simulink model "benchmarkss"  (Simulink 7.9)
settings: Solver=ode15s  SolverMode=SingleTasking  StartTime=0.0  StopTime=150  FixedStep=0.01  RelTol=1e-5  AbsTol=1e-8
values from neighbouring files (symbols this model uses):
  Qin0 = 18446    [states.mat]
  Qintr = 16485.6074222    [states.mat]
  Qintrawstate = 0    [states.mat]
  Qintrintstate = -2014.39257785    [states.mat]
  SETTLERINIT = [12.501625291 18.1183173569 29.5480012161 69.0014901899 356.282470924 356.282470935 356.282470923 356.282470934 356.282470923 6399.29814462 30 30 ... (80 elements, 1x80)]    [states.mat]
  SO5awstate = 1160.56564631    [states.mat]
  SO5intstate = -1172.91424974    [states.mat]
  XINIT1 = [30 3.24393684526 1149.16825994 98.6028769556 2552.10953282 151.672059002 446.924884063 0.00769641505704 3.51326345277 11.8311788245 1.36208895519 6.17753127623 ... (15 elements, 1x15)]    [states.mat]
  XINIT2 = [30 1.67067015162 1149.16825989 91.7032143318 2552.3710778 151.530315219 448.083853672 6.02712619456e-05 0.999999999994 12.5481626127 0.788988192675 5.95370072728 ... (15 elements, 1x15)]    [states.mat]
  XINIT3 = [30 1.21951265626 1149.16825982 69.6593696369 2560.20249467 152.687333601 449.633569515 1.63502587307 6.22889933341 7.31965726619 0.830700760805 4.71313752465 ... (15 elements, 1x15)]    [states.mat]
  XINIT4 = [30 0.973258200881 1149.16825975 54.4484250888 2563.31043926 153.710829707 451.185250351 2.47452269527 11.0693154946 2.7825370247 0.752763867168 3.84029820267 ... (15 elements, 1x15)]    [states.mat]
  XINIT5 = [30 0.808007806448 1149.16825967 44.4828030813 2562.85141224 154.163014752 452.736701239 2.00000000001 13.5243173117 0.671926961295 0.66449772338 3.26046452657 ... (15 elements, 1x15)]    [states.mat]
  XINITDELAY = [1601328.22267 1310222.01149 61339852.2439 6069822.46695 135212240.468 8102155.18077 23793923.6941 69863.2148447 472426.142984 605627.248842 151411.673606 366699.347571 ... (15 elements, 1x15)]    [states.mat]
undefined symbols (not defined in the file or in its folder): carb1, carb2, carb3, carb4, carb5, DIM, Kfeedforward, KLa1, KLa2, KLa3, KLa4, KLa5_max, KLa5offset, KQintr, KSO5, LAYER, MODELTYPE, PAR1, PAR2, PAR3, PAR4, PAR5, Qffref, Qintr_max, Qintroffset, QintrT, SETTLERPAR, SNO2ref, SO5ref, SOSAT1, SOSAT2, SOSAT3, SOSAT4, SOSAT5, T, TiQintr, TiSO5, TtQintr, TtSO5, useantiwindupQintr, useantiwindupSO5, VOL1, VOL2, VOL3, VOL4, VOL5
libraries: simulink x3
settings Model: Creator=ielulf  LastModifiedBy=SCUT2  ExtModeTrigMode=oneshot  ExtModeArmWhenConnect=off  ExtModeAutoUpdateStatusClock=off
settings DataIOCC: LimitDataPoints=off  SaveOutput=off  TimeSaveName=t  SignalLoggingName=sigsOut  OutputTimes=[143:(1/96):150]
settings OptimizationCC: BlockReduction=off  BooleanDataType=off  InitFltsAndDblsToZero=on
settings DebuggingCC: AlgebraicLoopMsg=none  SaveWithParameterizedLinksMsg=none  SignalResolutionControl=TryResolveAllWithWarning  SolverPrmCheckMsg=none  InheritedTsInSrcMsg=none  MultiTaskDSMMsg=warning  MultiTaskCondExecSysMsg=none  FcnCallInpInsideContextMsg=Use local settings  UnconnectedOutputMsg=none  StrictBusMsg=None
settings HardwareCC: TargetUnknown=on
settings RTWCC: TemplateMakefile=grt_unix.tmf  IncludeERTFirstTime=on
settings GRTTargetCC: TargetFcnLib=ansi_tfl_tmw.mat  CombineOutputUpdateFcns=off  GRTInterface=on

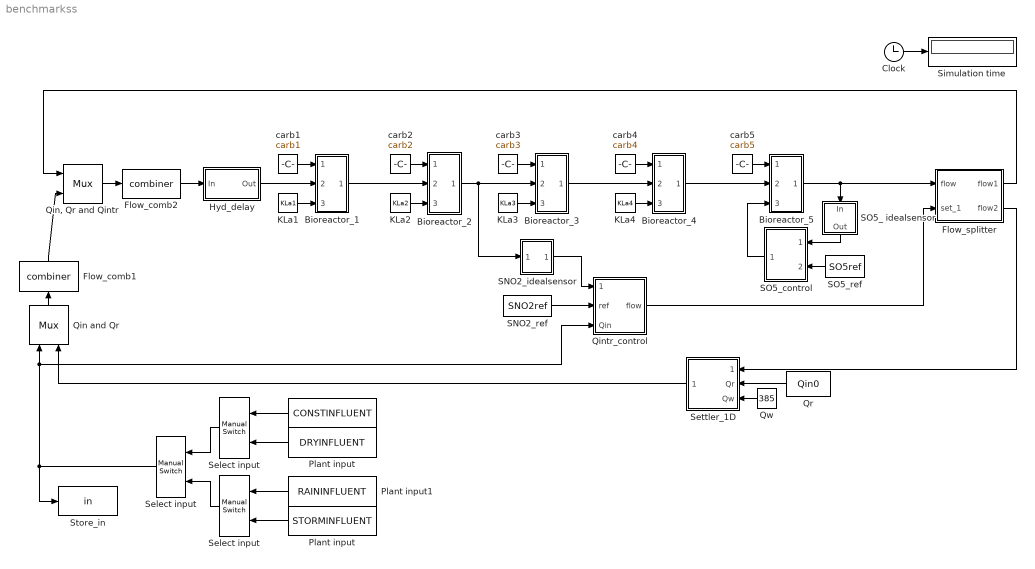
== system benchmarkss ==
  " " : FromWorkspace  VariableName=CONSTINFLUENT  OutputAfterFinalValue=Holding final value
  " Select input" : simulink/Signal Routing/Manual Switch  sw=1  action=0  varsize=off
  Bioreactor_1 : Subsystem
  Bioreactor_2 : Subsystem
  Bioreactor_3 : Subsystem
  Bioreactor_4 : Subsystem
  Bioreactor_5 : Subsystem
  Clock : Clock
  Flow_comb1 : S-Function  FunctionName=combiner  EnableBusSupport=off
  Flow_comb2 : S-Function  FunctionName=combiner  EnableBusSupport=off
  Flow_splitter : Subsystem
  Hyd_delay : Subsystem
  KLa1 : Constant  Value=KLa1
  KLa2 : Constant  Value=KLa2
  KLa3 : Constant  Value=KLa3
  KLa4 : Constant  Value=KLa4
  Plant input : FromWorkspace  VariableName=DRYINFLUENT  OutputAfterFinalValue=Holding final value
  "Plant input " : FromWorkspace  VariableName=STORMINFLUENT  OutputAfterFinalValue=Holding final value
  Plant input1 : FromWorkspace  VariableName=RAININFLUENT  OutputAfterFinalValue=Holding final value
  Qin and Qr : Mux  Inputs=2
  "Qin, Qr and Qintr" : Mux  Inputs=2
  Qintr_control : Subsystem
  Qr : Constant  Value=Qin0
  Qw : Constant  Value=385
  SNO2_idealsensor : Subsystem
  SNO2_ref : Constant  Value=SNO2ref
  SO5_ idealsensor : Subsystem
  SO5_control : Subsystem
  SO5_ref : Constant  Value=SO5ref
  Select input : simulink/Signal Routing/Manual Switch  sw=1  action=0  varsize=off
  "Select input " : simulink/Signal Routing/Manual Switch  sw=0  action=0  varsize=off
  Settler_1D : Subsystem
  Simulation time : Display
  Store_in : ToWorkspace  VariableName=in  SampleTime=-1
  carb1 : Constant  Value=carb1
  carb2 : Constant  Value=carb2
  carb3 : Constant  Value=carb3
  carb4 : Constant  Value=carb4
  carb5 : Constant  Value=carb5
  wires:
  Qin and Qr/1 -> Flow_comb1/1
  Flow_comb1/1 -> "Qin, Qr and Qintr"/2
  "Qin, Qr and Qintr"/1 -> Flow_comb2/1
  Flow_splitter/1(flow1) -> "Qin, Qr and Qintr"/1
  Settler_1D/1(output) -> Qin and Qr/2
  Qw/1 -> Settler_1D/3(Qw)
  Flow_splitter/2(flow2) -> Settler_1D/1(feed)
  Qr/1 -> Settler_1D/2(Qr)
  Bioreactor_5/1(out) -> Flow_splitter/1(flow), SO5_ idealsensor/1(In)
  Flow_comb2/1 -> Hyd_delay/1(In)
  Clock/1 -> Simulation time/1
  Plant input/1 -> Select input/2
  " "/1 -> Select input/1
  Hyd_delay/1(Out) -> Bioreactor_1/2(in)
  carb1/1 -> Bioreactor_1/1(carb)
  KLa1/1 -> Bioreactor_1/3(KLa)
  Bioreactor_1/1(out) -> Bioreactor_2/2(in)
  KLa2/1 -> Bioreactor_2/3(KLa)
  carb2/1 -> Bioreactor_2/1(carb)
  Bioreactor_2/1(out) -> Bioreactor_3/2(in), SNO2_idealsensor/1(In)
  KLa3/1 -> Bioreactor_3/3(KLa)
  carb3/1 -> Bioreactor_3/1(carb)
  Bioreactor_3/1(out) -> Bioreactor_4/2(in)
  KLa4/1 -> Bioreactor_4/3(KLa)
  carb4/1 -> Bioreactor_4/1(carb)
  Bioreactor_4/1(out) -> Bioreactor_5/2(in)
  carb5/1 -> Bioreactor_5/1(carb)
  Plant input1/1 -> "Select input "/1
  "Plant input "/1 -> "Select input "/2
  Select input/1 -> " Select input"/1
  "Select input "/1 -> " Select input"/2
  " Select input"/1 -> Store_in/1, Qin and Qr/1, Qintr_control/3(Qin)
  SNO2_ref/1 -> Qintr_control/2(ref)
  SNO2_idealsensor/1(Out) -> Qintr_control/1(meas)
  Qintr_control/1(flow) -> Flow_splitter/2(set_1)
  SO5_ref/1 -> SO5_control/2(O2_ref)
  SO5_control/1(KLa) -> Bioreactor_5/3(KLa)
  SO5_ idealsensor/1(Out) -> SO5_control/1(O2_meas)

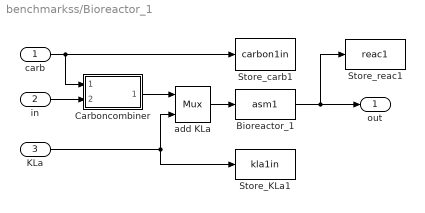
== system benchmarkss/Bioreactor_1 ==
  carb : Inport
  in : Inport  Port=2
  KLa : Inport  Port=3
  Bioreactor_1 : S-Function  FunctionName=asm1  Parameters=XINIT1,PAR1,VOL1,SOSAT1  EnableBusSupport=off
  Carboncombiner : Subsystem
  Store_KLa1 : ToWorkspace  VariableName=kla1in  SampleTime=-1
  Store_carb1 : ToWorkspace  VariableName=carbon1in  SampleTime=-1
  Store_reac1 : ToWorkspace  VariableName=reac1  SampleTime=-1
  add KLa : Mux  Inputs=2
  out : Outport
  wires:
  add KLa/1 -> Bioreactor_1/1
  Bioreactor_1/1 -> out/1, Store_reac1/1
  Carboncombiner/1(Output) -> add KLa/1
  carb/1 -> Store_carb1/1, Carboncombiner/1(C_flow)
  in/1 -> Carboncombiner/2(Input)
  KLa/1 -> add KLa/2, Store_KLa1/1

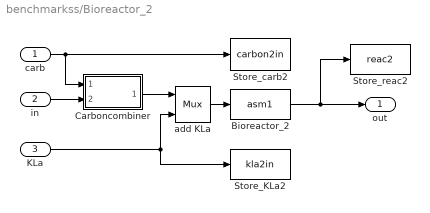
== system benchmarkss/Bioreactor_2 ==
  carb : Inport
  in : Inport  Port=2
  KLa : Inport  Port=3
  Bioreactor_2 : S-Function  FunctionName=asm1  Parameters=XINIT2,PAR2,VOL2,SOSAT2  EnableBusSupport=off
  Carboncombiner : Subsystem
  Store_KLa2 : ToWorkspace  VariableName=kla2in  SampleTime=-1
  Store_carb2 : ToWorkspace  VariableName=carbon2in  SampleTime=-1
  Store_reac2 : ToWorkspace  VariableName=reac2  SampleTime=-1
  add KLa : Mux  Inputs=2
  out : Outport
  wires:
  Bioreactor_2/1 -> out/1, Store_reac2/1
  add KLa/1 -> Bioreactor_2/1
  Carboncombiner/1(Output) -> add KLa/1
  carb/1 -> Carboncombiner/1(C_flow), Store_carb2/1
  in/1 -> Carboncombiner/2(Input)
  KLa/1 -> add KLa/2, Store_KLa2/1

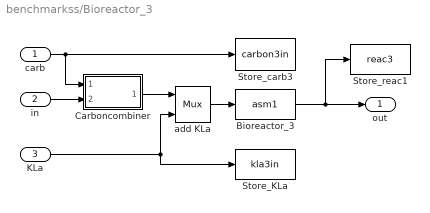
== system benchmarkss/Bioreactor_3 ==
  carb : Inport
  in : Inport  Port=2
  KLa : Inport  Port=3
  Bioreactor_3 : S-Function  FunctionName=asm1  Parameters=XINIT3,PAR3,VOL3,SOSAT3  EnableBusSupport=off
  Carboncombiner : Subsystem
  Store_KLa : ToWorkspace  VariableName=kla3in  SampleTime=-1
  Store_carb3 : ToWorkspace  VariableName=carbon3in  SampleTime=-1
  Store_reac1 : ToWorkspace  VariableName=reac3  SampleTime=-1
  add KLa : Mux  Inputs=2
  out : Outport
  wires:
  Bioreactor_3/1 -> out/1, Store_reac1/1
  add KLa/1 -> Bioreactor_3/1
  Carboncombiner/1(Output) -> add KLa/1
  carb/1 -> Carboncombiner/1(C_flow), Store_carb3/1
  in/1 -> Carboncombiner/2(Input)
  KLa/1 -> add KLa/2, Store_KLa/1

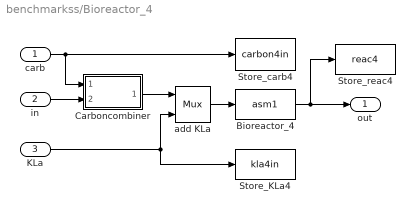
== system benchmarkss/Bioreactor_4 ==
  carb : Inport
  in : Inport  Port=2
  KLa : Inport  Port=3
  Bioreactor_4 : S-Function  FunctionName=asm1  Parameters=XINIT4,PAR4,VOL4,SOSAT4  EnableBusSupport=off
  Carboncombiner : Subsystem
  Store_KLa4 : ToWorkspace  VariableName=kla4in  SampleTime=-1
  Store_carb4 : ToWorkspace  VariableName=carbon4in  SampleTime=-1
  Store_reac4 : ToWorkspace  VariableName=reac4  SampleTime=-1
  add KLa : Mux  Inputs=2
  out : Outport
  wires:
  Bioreactor_4/1 -> out/1, Store_reac4/1
  add KLa/1 -> Bioreactor_4/1
  Carboncombiner/1(Output) -> add KLa/1
  carb/1 -> Carboncombiner/1(C_flow), Store_carb4/1
  in/1 -> Carboncombiner/2(Input)
  KLa/1 -> add KLa/2, Store_KLa4/1

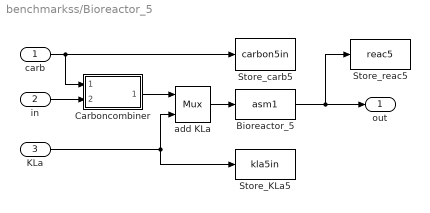
== system benchmarkss/Bioreactor_5 ==
  carb : Inport
  in : Inport  Port=2
  KLa : Inport  Port=3
  Bioreactor_5 : S-Function  FunctionName=asm1  Parameters=XINIT5,PAR5,VOL5,SOSAT5  EnableBusSupport=off
  Carboncombiner : Subsystem
  Store_KLa5 : ToWorkspace  VariableName=kla5in  SampleTime=-1
  Store_carb5 : ToWorkspace  VariableName=carbon5in  SampleTime=-1
  Store_reac5 : ToWorkspace  VariableName=reac5  SampleTime=-1
  add KLa : Mux  Inputs=2
  out : Outport
  wires:
  Bioreactor_5/1 -> out/1, Store_reac5/1
  add KLa/1 -> Bioreactor_5/1
  Carboncombiner/1(Output) -> add KLa/1
  carb/1 -> Carboncombiner/1(C_flow), Store_carb5/1
  in/1 -> Carboncombiner/2(Input)
  KLa/1 -> add KLa/2, Store_KLa5/1

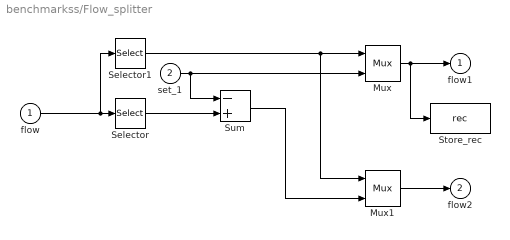
== system benchmarkss/Flow_splitter ==
  flow : Inport
  set_1 : Inport  Port=2
  Mux : Mux  Inputs=2
  Mux1 : Mux  Inputs=2
  Selector : Selector  InputPortWidth=15  IndexOptions=Index vector (dialog)  Indices=[15]  OutputSizes=1
  Selector1 : Selector  InputPortWidth=15  IndexOptions=Index vector (dialog)  Indices=[1 2 3 4 5 6 7 8 9 10 11 12 13 14]  OutputSizes=1
  Store_rec : ToWorkspace  VariableName=rec  SampleTime=-1
  Sum : Sum  Inputs=-+  SaturateOnIntegerOverflow=on  InputSameDT=on  OutDataTypeStr=Inherit: Same as first input
  flow1 : Outport
  flow2 : Outport  Port=2
  wires:
  flow/1 -> Selector1/1, Selector/1
  Mux/1 -> flow1/1, Store_rec/1
  Mux1/1 -> flow2/1
  set_1/1 -> Mux/2, Sum/1
  Selector/1 -> Sum/2
  Sum/1 -> Mux1/2
  Selector1/1 -> Mux/1, Mux1/1

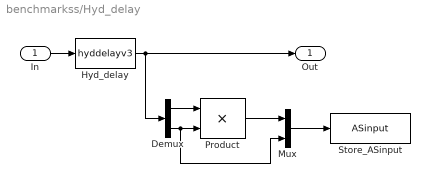
== system benchmarkss/Hyd_delay ==
  In : Inport
  Demux : Demux  Outputs=[14,1]
  Hyd_delay : S-Function  FunctionName=hyddelayv3  Parameters=XINITDELAY,PAR1,T  EnableBusSupport=off
  Mux : Mux  Inputs=2
  Product : Product  SaturateOnIntegerOverflow=on  OutDataTypeStr=Inherit: Same as first input
  Store_ASinput : ToWorkspace  VariableName=ASinput  SampleTime=-1
  Out : Outport
  wires:
  In/1 -> Hyd_delay/1
  Hyd_delay/1 -> Out/1, Demux/1
  Demux/1 -> Product/1
  Demux/2 -> Product/2, Mux/2
  Product/1 -> Mux/1
  Mux/1 -> Store_ASinput/1

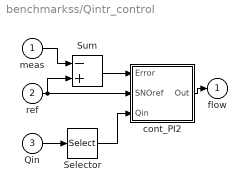
== system benchmarkss/Qintr_control ==
  meas : Inport
  ref : Inport  Port=2
  Qin : Inport  Port=3
  Selector : Selector  InputPortWidth=15  IndexOptions=Index vector (dialog)  Indices=[15]  OutputSizes=1
  Sum : Sum  Inputs=-+  SaturateOnIntegerOverflow=on  InputSameDT=on  OutDataTypeStr=Inherit: Same as first input
  cont_PI2 : Subsystem
  flow : Outport
  wires:
  Selector/1 -> cont_PI2/3(Qin)
  ref/1 -> cont_PI2/2(SNOref), Sum/2
  Qin/1 -> Selector/1
  cont_PI2/1(Out) -> flow/1
  Sum/1 -> cont_PI2/1(Error)
  meas/1 -> Sum/1

== system benchmarkss/SNO2_idealsensor ==
  In : Inport
  Mux : Mux  Inputs=6
  Selector : Selector  InputPortWidth=15  IndexOptions=Index vector (dialog)  Indices=[9]  OutputSizes=1
  To Workspace : ToWorkspace  VariableName=SNO2sensor  SampleTime=-1
  Out : Outport
  wires:
  Selector/1 -> Mux/3, Mux/4, Out/1, Mux/5, Mux/6, Mux/2, Mux/1
  In/1 -> Selector/1
  Mux/1 -> To Workspace/1

== system benchmarkss/SO5_ idealsensor ==
  In : Inport
  Mux : Mux  Inputs=6
  Selector : Selector  InputPortWidth=15  IndexOptions=Index vector (dialog)  Indices=[8]  OutputSizes=1
  To Workspace : ToWorkspace  VariableName=SO5sensor  SampleTime=-1
  Out : Outport
  wires:
  Selector/1 -> Mux/3, Mux/4, Out/1, Mux/5, Mux/6, Mux/2, Mux/1
  In/1 -> Selector/1
  Mux/1 -> To Workspace/1

== system benchmarkss/SO5_control ==
  O2_meas : Inport
  O2_ref : Inport  Port=2
  Sum : Sum  Inputs=-+  SaturateOnIntegerOverflow=on  InputSameDT=on  OutDataTypeStr=Inherit: Same as first input
  cont_PI : Subsystem
  KLa : Outport
  wires:
  O2_meas/1 -> Sum/1
  cont_PI/1(Out) -> KLa/1
  O2_ref/1 -> Sum/2
  Sum/1 -> cont_PI/1(In)

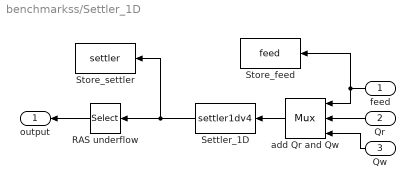
== system benchmarkss/Settler_1D ==
  feed : Inport
  Qr : Inport  Port=2
  Qw : Inport  Port=3
  RAS underflow : Selector  InputPortWidth=113  IndexOptions=Index vector (dialog)  Indices=[1 2 3 4 5 6 7 8 9 10 11 12 13 14 15]  OutputSizes=1
  Settler_1D : S-Function  FunctionName=settler1dv4  Parameters=SETTLERINIT,SETTLERPAR,DIM,LAYER,MODELTYPE  EnableBusSupport=off
  Store_feed : ToWorkspace  VariableName=feed  SampleTime=-1
  Store_settler : ToWorkspace  VariableName=settler  SampleTime=-1
  add Qr and Qw : Mux  Inputs=3
  output : Outport
  wires:
  add Qr and Qw/1 -> Settler_1D/1
  Qr/1 -> add Qr and Qw/2
  Qw/1 -> add Qr and Qw/3
  feed/1 -> add Qr and Qw/1, Store_feed/1
  RAS underflow/1 -> output/1
  Settler_1D/1 -> RAS underflow/1, Store_settler/1

== system benchmarkss/Bioreactor_1/Carboncombiner ==
  C_flow : Inport
  Input : Inport  Port=2
  Carboncombiner : S-Function  FunctionName=carboncombiner  Parameters=CARBONSOURCECONC  EnableBusSupport=off
  Mux : Mux  Inputs=2
  Output : Outport
  wires:
  C_flow/1 -> Mux/1
  Mux/1 -> Carboncombiner/1
  Carboncombiner/1 -> Output/1
  Input/1 -> Mux/2

== system benchmarkss/Bioreactor_2/Carboncombiner ==
  C_flow : Inport
  Input : Inport  Port=2
  Carboncombiner : S-Function  FunctionName=carboncombiner  Parameters=CARBONSOURCECONC  EnableBusSupport=off
  Mux : Mux  Inputs=2
  Output : Outport
  wires:
  Input/1 -> Mux/2
  Carboncombiner/1 -> Output/1
  Mux/1 -> Carboncombiner/1
  C_flow/1 -> Mux/1

== system benchmarkss/Bioreactor_3/Carboncombiner ==
  C_flow : Inport
  Input : Inport  Port=2
  Carboncombiner : S-Function  FunctionName=carboncombiner  Parameters=CARBONSOURCECONC  EnableBusSupport=off
  Mux : Mux  Inputs=2
  Output : Outport
  wires:
  Input/1 -> Mux/2
  Carboncombiner/1 -> Output/1
  Mux/1 -> Carboncombiner/1
  C_flow/1 -> Mux/1

== system benchmarkss/Bioreactor_4/Carboncombiner ==
  C_flow : Inport
  Input : Inport  Port=2
  Carboncombiner : S-Function  FunctionName=carboncombiner  Parameters=CARBONSOURCECONC  EnableBusSupport=off
  Mux : Mux  Inputs=2
  Output : Outport
  wires:
  Input/1 -> Mux/2
  Carboncombiner/1 -> Output/1
  Mux/1 -> Carboncombiner/1
  C_flow/1 -> Mux/1

== system benchmarkss/Bioreactor_5/Carboncombiner ==
  C_flow : Inport
  Input : Inport  Port=2
  Carboncombiner : S-Function  FunctionName=carboncombiner  Parameters=CARBONSOURCECONC  EnableBusSupport=off
  Mux : Mux  Inputs=2
  Output : Outport
  wires:
  Input/1 -> Mux/2
  Carboncombiner/1 -> Output/1
  Mux/1 -> Carboncombiner/1
  C_flow/1 -> Mux/1

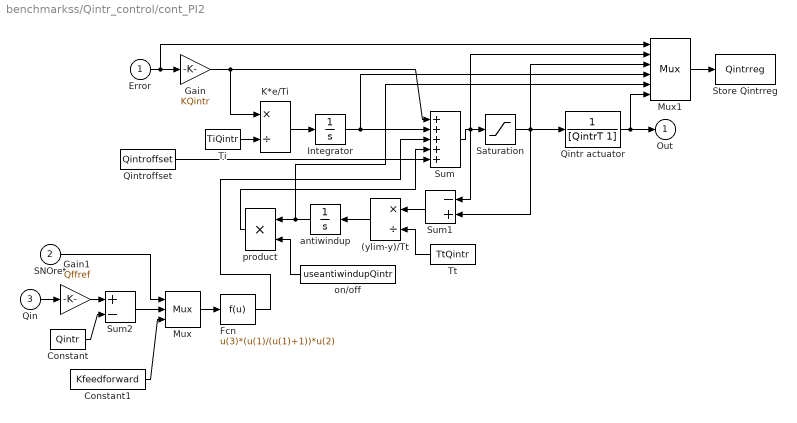
== system benchmarkss/Qintr_control/cont_PI2 ==
  Error : Inport
  SNOref : Inport  Port=2
  Qin : Inport  Port=3
  (ylim-y)/Tt : Product  Inputs=*/  SaturateOnIntegerOverflow=on  InputSameDT=on  OutDataTypeStr=Inherit: Same as first input
  Constant : Constant  Value=Qintr
  Constant1 : Constant  Value=Kfeedforward
  Fcn : Fcn  Expr=u(3)*(u(1)/(u(1)+1))*u(2)
  Gain : Gain  Gain=KQintr  SaturateOnIntegerOverflow=on  OutDataTypeStr=Inherit: Same as input  ParamDataTypeStr=Inherit: Same as input
  Gain1 : Gain  Gain=Qffref  SaturateOnIntegerOverflow=on  OutDataTypeStr=Inherit: Same as input  ParamDataTypeStr=Inherit: Same as input
  Integrator : Integrator  InitialCondition=Qintrintstate
  K*e/Ti : Product  Inputs=*/  SaturateOnIntegerOverflow=on  InputSameDT=on  OutDataTypeStr=Inherit: Same as first input
  Mux : Mux  Inputs=3
  Mux1 : Mux  Inputs=6
  Qintr actuator : TransferFcn  Denominator=[QintrT 1]
  Qintroffset : Constant  Value=Qintroffset
  Saturation : Saturate  UpperLimit=Qintr_max  LowerLimit=0
  Store Qintrreg : ToWorkspace  VariableName=Qintrreg  SampleTime=-1
  Sum : Sum  Inputs=+++++  SaturateOnIntegerOverflow=on  InputSameDT=on  OutDataTypeStr=Inherit: Same as first input
  Sum1 : Sum  Inputs=-+  SaturateOnIntegerOverflow=on  InputSameDT=on  OutDataTypeStr=Inherit: Same as first input
  Sum2 : Sum  Inputs=+-  SaturateOnIntegerOverflow=on  InputSameDT=on  OutDataTypeStr=Inherit: Same as first input
  Ti : Constant  Value=TiQintr
  Tt : Constant  Value=TtQintr
  antiwindup : Integrator  InitialCondition=Qintrawstate
  on/off : Constant  Value=useantiwindupQintr
  product : Product  Inputs=**  SaturateOnIntegerOverflow=on  InputSameDT=on  OutDataTypeStr=Inherit: Same as first input
  Out : Outport
  wires:
  Qintroffset/1 -> Sum/5
  Gain1/1 -> Sum2/1
  Qin/1 -> Gain1/1
  Constant/1 -> Sum2/2
  antiwindup/1 -> Mux1/5, product/1
  Integrator/1 -> Mux1/4, Sum/2
  Fcn/1 -> Sum/3
  Mux/1 -> Fcn/1
  SNOref/1 -> Mux/1
  product/1 -> Sum/4
  K*e/Ti/1 -> Integrator/1
  Ti/1 -> K*e/Ti/2
  Gain/1 -> K*e/Ti/1, Sum/1
  Sum1/1 -> (ylim-y)/Tt/1
  Tt/1 -> (ylim-y)/Tt/2
  (ylim-y)/Tt/1 -> antiwindup/1
  Sum/1 -> Saturation/1, Sum1/1, Mux1/2
  Saturation/1 -> Sum1/2, Qintr actuator/1, Mux1/3
  Mux1/1 -> Store Qintrreg/1
  Error/1 -> Gain/1, Mux1/1
  on/off/1 -> product/2
  Constant1/1 -> Mux/3
  Sum2/1 -> Mux/2
  Qintr actuator/1 -> Out/1, Mux1/6

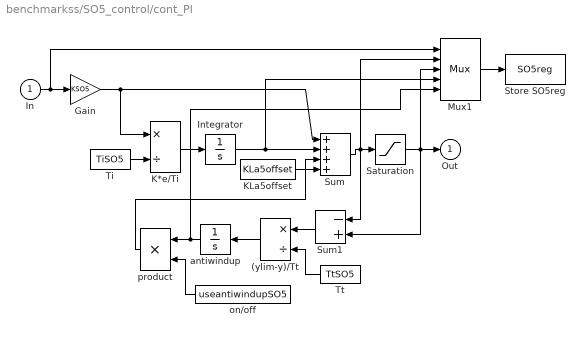
== system benchmarkss/SO5_control/cont_PI ==
  In : Inport
  (ylim-y)/Tt : Product  Inputs=*/  SaturateOnIntegerOverflow=on  InputSameDT=on  OutDataTypeStr=Inherit: Same as first input
  Gain : Gain  Gain=KSO5  SaturateOnIntegerOverflow=on  OutDataTypeStr=Inherit: Same as input  ParamDataTypeStr=Inherit: Same as input
  Integrator : Integrator  InitialCondition=SO5intstate
  K*e/Ti : Product  Inputs=*/  SaturateOnIntegerOverflow=on  InputSameDT=on  OutDataTypeStr=Inherit: Same as first input
  KLa5offset : Constant  Value=KLa5offset
  Mux1 : Mux  Inputs=5
  Saturation : Saturate  UpperLimit=KLa5_max  LowerLimit=0
  Store SO5reg : ToWorkspace  VariableName=SO5reg  SampleTime=-1
  Sum : Sum  Inputs=++++  SaturateOnIntegerOverflow=on  InputSameDT=on  OutDataTypeStr=Inherit: Same as first input
  Sum1 : Sum  Inputs=-+  SaturateOnIntegerOverflow=on  InputSameDT=on  OutDataTypeStr=Inherit: Same as first input
  Ti : Constant  Value=TiSO5
  Tt : Constant  Value=TtSO5
  antiwindup : Integrator  InitialCondition=SO5awstate
  on/off : Constant  Value=useantiwindupSO5
  product : Product  Inputs=**  SaturateOnIntegerOverflow=on  InputSameDT=on  OutDataTypeStr=Inherit: Same as first input
  Out : Outport
  wires:
  KLa5offset/1 -> Sum/4
  antiwindup/1 -> Mux1/5, product/1
  Integrator/1 -> Mux1/4, Sum/2
  Mux1/1 -> Store SO5reg/1
  Saturation/1 -> Mux1/3, Sum1/2, Out/1
  Sum/1 -> Mux1/2, Sum1/1, Saturation/1
  (ylim-y)/Tt/1 -> antiwindup/1
  Tt/1 -> (ylim-y)/Tt/2
  Sum1/1 -> (ylim-y)/Tt/1
  Gain/1 -> K*e/Ti/1, Sum/1
  Ti/1 -> K*e/Ti/2
  K*e/Ti/1 -> Integrator/1
  In/1 -> Gain/1, Mux1/1
  on/off/1 -> product/2
  product/1 -> Sum/3
